simulink model "MCSI_simulation_2024_HDL_Coder_test"  (R2021a)
settings: Solver=VariableStepAuto  StartTime=0.0  StopTime=5/cfg.fl  FixedStep=2.0833e-8  RelTol=1e-3
undefined symbols (not defined in the file or in its folder): cfg
libraries: spsIdealSwitchLib x18, simulink x12, hdlsllib x8, spsSeriesRLCBranchLib x7, spsCurrentMeasurementLib x4, commutil2 x3, spsMeanLib x2, spsThreePhaseSeriesRLCBranchLib x2, spsThreePhaseVIMeasurementLib x2, spsControlledCurrentSourceLib x1, spsGroundLib x1, spsThreePhaseProgrammableGeneratorLib x1
settings Model: Creator=Damian  LastModifiedBy=Damian
settings SimscapeCC: SimscapeLogType=all  SimscapeLogLimitData=off

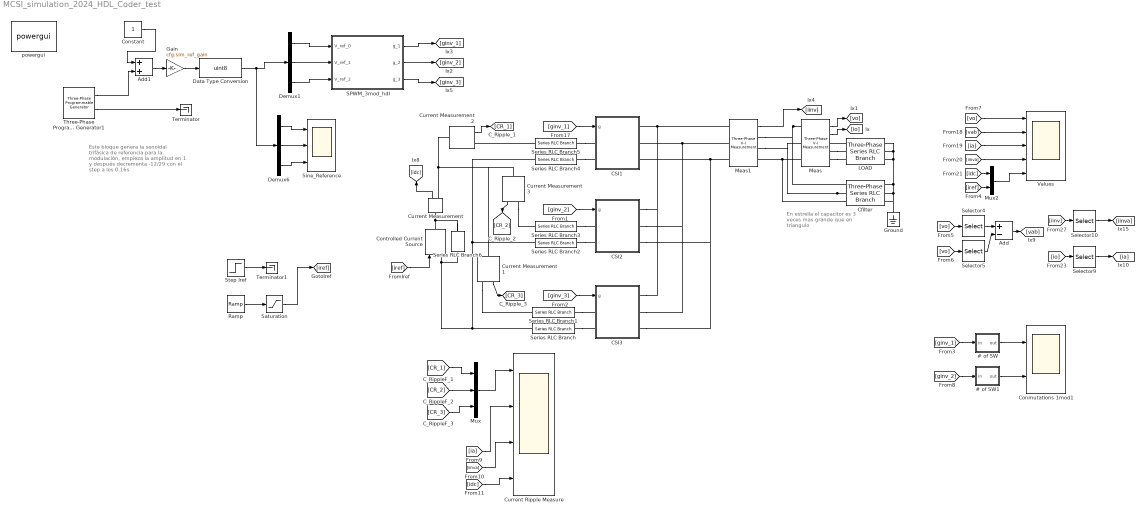
== system MCSI_simulation_2024_HDL_Coder_test ==
  note: Este bloque genera la senoidal
      | trifásica de referencia para la
      | modulación, empieza la amplitud
      | en 1 y después decrementa -12/29
      | con el step a los 0.16s
  note: En estrella el capacitor
      | es 3 veces mas grande
      | que en triangulo
  # of SW : Subsystem
  # of SW1 : Subsystem
  Add : Sum  Inputs=+-
  Add1 : Sum
  CSI1 : Subsystem
  CSI2 : Subsystem
  CSI3 : Subsystem
  Cfilter : spsThreePhaseSeriesRLCBranchLib/Three-Phase Series RLC Branch  LConnTagsString=A|B|C  RConnTagsString=A|B|C  BranchType=C  Resistance=1  Inductance=cfg.c  Capacitance=cfg.c  Measurements=None
  Conmutations 1mod1 : Scope  NumInputPorts=2
  Constant : Constant
  Controlled Current Source : spsControlledCurrentSourceLib/Controlled Current Source  Initialize=on  Source_Type=AC  Amplitude=0  Phase=0  Frequency=0  Measurements=None
  Current Measurement{,1..3} (4 alike) : spsCurrentMeasurementLib/Current Measurement  PhasorSimulation=off  OutputType=Complex  PSBequivalent=0
  Current Ripple Measure : Scope  NumInputPorts=4
  Data Type Conversion : DataTypeConversion  OutDataTypeStr=uint8
  Demux1 : Demux  Outputs=3
  Demux6 : Demux  Outputs=3
  Gain : Gain  Gain=cfg.sim_ref_gain
  Ground : spsGroundLib/Ground  LConnTagsString=a
  LOAD : spsThreePhaseSeriesRLCBranchLib/Three-Phase Series RLC Branch  LConnTagsString=A|B|C  RConnTagsString=A|B|C  BranchType=RL  Resistance=cfg.r  Inductance=cfg.l  Capacitance=1e-6  Measurements=None
  Meas : spsThreePhaseVIMeasurementLib/Three-Phase V-I Measurement  VoltageMeasurement=phase-to-ground  SetLabelV=off  LabelV=Vabc  Vpu=off  VpuLL=off  CurrentMeasurement=yes  SetLabelI=off  LabelI=Iabc  Ipu=off  Pbase=100e6  Vbase=500e3  OutputType=Complex  PhasorSimulation=off  PSBequivalent=0
  Meas1 : spsThreePhaseVIMeasurementLib/Three-Phase V-I Measurement  VoltageMeasurement=no  SetLabelV=off  LabelV=Vabc  Vpu=off  VpuLL=off  CurrentMeasurement=yes  SetLabelI=off  LabelI=Iabc  Ipu=off  Pbase=100e6  Vbase=500e3  OutputType=Complex  PhasorSimulation=off  PSBequivalent=0
  Mux : Mux  Inputs=3
  Mux2 : Mux  Inputs=2
  Ramp : simulink/Sources/Ramp  slope=cfg.iref/cfg.cs_soft_start_time  start=0  InitialOutput=0
  SPWM_3mod_hdl : Subsystem
  Saturation : Saturate  UpperLimit=10  LowerLimit=0
  Selector10 : Selector  InputPortWidth=3  IndexOptions=Index vector (dialog)  Indices=1  OutputSizes=1
  Selector4 : Selector  InputPortWidth=3  IndexOptions=Index vector (dialog)  Indices=1  OutputSizes=1
  Selector5 : Selector  InputPortWidth=3  IndexOptions=Index vector (dialog)  Indices=2  OutputSizes=1
  Selector9 : Selector  InputPortWidth=3  IndexOptions=Index vector (dialog)  Indices=1  OutputSizes=1
  Series RLC Branch{,1..5} (6 alike) : spsSeriesRLCBranchLib/Series RLC Branch  LConnTagsString=__new0  RConnTagsString=__new0  BranchType=L  Resistance=1  Inductance=cfg.sharing_L  SetiL0=off  InitialCurrent=0  Capacitance=1e-6  Setx0=off  InitialVoltage=0  Measurements=None
  Series RLC Branch6 : spsSeriesRLCBranchLib/Series RLC Branch  LConnTagsString=__new0  RConnTagsString=__new0  BranchType=R  Resistance=1E5  Inductance=cfg.sharing_L  SetiL0=off  InitialCurrent=0  Capacitance=1e-6  Setx0=off  InitialVoltage=0  Measurements=None
  Sine_Reference : Scope  NumInputPorts=3
  Step Iref : Step  Time=12/cfg.fl  Before=cfg.iref  After=0.6*cfg.iref  SampleTime=cfg.ts
  Terminator : Terminator
  Terminator1 : Terminator
  Three-Phase Programmable Generator1 : spsThreePhaseProgrammableGeneratorLib/Three-Phase Programmable Generator  Par_Vps=[1,-30, cfg.fl]  VariationEntity=None  VariationType=Step  VariationStep=-12/29  VariationRate=10  VariationMag=0.3  VariationFreq=2  Par_Timing_Variation="[8/cfg.fl  10]"  SinglePhase=on  Yampli=[1 0.2 1.2 1.0]  Xtime=[0 0.1 0.15 0.2]  HarmonicGeneration=off  Par_HarmoA="[3  5  -25 0]"  Par_HarmoB="[5  10  35  2]"  Par_Timing_Harmo="[ 0.05  99]"  Ts=cfg.ts
      settings: SourceProductBaseCode=PS
  Values : Scope  NumInputPorts=5
  powergui : spspowerguiLib/powergui  Priority=1  SimulationMode=Discrete  SampleTime=cfg.ts  frequency=60  Iterations=50  frequencyindice=0  Pbase=100e6  ErrMax=1e-4  UnitsV=kV  UnitsW=MW  buscounter=0  FunctionMessages=off  echomessages=off  EnableUseOfTLC=off  CurrentSourceSwitches=off  DisableSnubberDevices=off  DisableRonSwitches=off  DisableVfSwitches=off  DisplayEquations=off  AutomaticDiscreteSolvers=off  SolverType=Backward Euler  Interpol=off  ExternalGateDelay=off  methode=off  Ts=0  x0status=blocks  SPID=off  SwTol=0  HookPort=off  NonlinearTolerance=1e-4  nMaxIteration=100  ContinueOnMaxIteration=off  RestoreLinks=warning  ResistiveCurrentMeasurement=off  Frange=[0:2:500]  Ylog=off  Xlog=on  ShowGrid=off  save=off  variable=ZData  structure=one_mod_model  ZoomFFT=off  StartTime=0.12  cycles=1  DisplayStyle=1  fundamental=50  FreqAxis=off  MaxFrequency=1000  frequencyindicesteady=1  RmsSteady=1  display=off
  wires:
  [iref] -> Controlled Current Source/1
  Current Measurement/1 -> [idc]
  Three-Phase Programmable Generator1/2 -> Terminator/1
  Three-Phase Programmable Generator1/1 -> Add1/2
  Demux6/3 -> Sine_Reference/3
  Demux6/2 -> Sine_Reference/2
  Demux6/1 -> Sine_Reference/1
  [ginv_1] -> CSI1/1(g)
  Meas/1 -> [vo]
  Meas/2 -> [io]
  Meas1/1 -> [iinv]
  [iref] -> Mux2/2
  [idc] -> Mux2/1
  Mux2/1 -> Values/5
  [vo] -> Values/1
  [iinva] -> Values/4
  [ia] -> Values/3
  [vab] -> Values/2
  [vo] -> Selector4/1
  [vo] -> Selector5/1
  Selector4/1 -> Add/1
  Selector5/1 -> Add/2
  Add/1 -> [vab]
  [iinv] -> Selector10/1
  [io] -> Selector9/1
  Selector10/1 -> [iinva]
  Selector9/1 -> [ia]
  [ginv_2] -> CSI2/1(g)
  [ginv_3] -> CSI3/1(g)
  [ginv_1] -> # of SW/1(in)
  # of SW/1(out) -> Conmutations 1mod1/1
  # of SW1/1(out) -> Conmutations 1mod1/2
  [ginv_2] -> # of SW1/1(in)
  Saturation/1 -> [iref]
  Ramp/1 -> Saturation/1
  Step Iref/1 -> Terminator1/1
  Current Measurement2/1 -> [CR_1]
  Current Measurement3/1 -> [CR_2]
  Current Measurement1/1 -> [CR_3]
  [ia] -> Current Ripple Measure/2
  [iinva] -> Current Ripple Measure/3
  [idc] -> Current Ripple Measure/4
  [CR_1] -> Mux/1
  [CR_2] -> Mux/2
  [CR_3] -> Mux/3
  Mux/1 -> Current Ripple Measure/1
  Constant/1 -> Add1/1
  Add1/1 -> Gain/1
  Gain/1 -> Data Type Conversion/1
  Data Type Conversion/1 -> Demux6/1, Demux1/1
  Demux1/3 -> SPWM_3mod_hdl/3(V_ref_2)
  Demux1/2 -> SPWM_3mod_hdl/2(V_ref_1)
  Demux1/1 -> SPWM_3mod_hdl/1(V_ref_0)
  SPWM_3mod_hdl/1(g_1) -> [ginv_1]
  SPWM_3mod_hdl/2(g_2) -> [ginv_2]
  SPWM_3mod_hdl/3(g_3) -> [ginv_3]
  connections:
  Current Measurement/LConn1 -- Series RLC Branch6/LConn1 -- Controlled Current Source/RConn1
  Meas/LConn3 -- Cfilter/LConn3 -- Meas1/RConn3
  Meas/LConn1 -- Meas1/RConn1 -- Cfilter/LConn1
  LOAD/RConn2 -- LOAD/RConn1 -- LOAD/RConn3 -- Cfilter/RConn1 -- Cfilter/RConn2 -- Cfilter/RConn3 -- Ground/LConn1
  Cfilter/LConn2 -- Meas1/RConn2 -- Meas/LConn2
  LOAD/LConn1 -- Meas/RConn1
  Meas/RConn2 -- LOAD/LConn2
  Meas/RConn3 -- LOAD/LConn3
  Meas1/LConn1 -- CSI3/RConn1 -- CSI2/RConn1 -- CSI1/RConn1
  Meas1/LConn2 -- CSI3/RConn2 -- CSI2/RConn2 -- CSI1/RConn2
  Meas1/LConn3 -- CSI3/RConn3 -- CSI2/RConn3 -- CSI1/RConn3
  Series RLC Branch4/RConn1 -- CSI1/LConn2
  Series RLC Branch5/RConn1 -- CSI1/LConn1
  Series RLC Branch3/RConn1 -- CSI2/LConn1
  Series RLC Branch2/RConn1 -- CSI2/LConn2
  Series RLC Branch1/RConn1 -- CSI3/LConn1
  Series RLC Branch/RConn1 -- CSI3/LConn2
  Controlled Current Source/LConn1 -- Series RLC Branch/LConn1 -- Series RLC Branch2/LConn1 -- Series RLC Branch4/LConn1 -- Series RLC Branch6/RConn1
  Current Measurement3/RConn1 -- Series RLC Branch3/LConn1
  Current Measurement2/LConn1 -- Current Measurement3/LConn1 -- Current Measurement1/LConn1 -- Current Measurement/RConn1
  Current Measurement1/RConn1 -- Series RLC Branch1/LConn1
  Series RLC Branch5/LConn1 -- Current Measurement2/RConn1

== system MCSI_simulation_2024_HDL_Coder_test/# of SW ==
  in : Inport
  Data Type Conversion : DataTypeConversion
  Detect Change : simulink/Logic and Bit Operations/Detect Change  vinit=0  OutDataTypeStr=boolean
  Divide : Product  Inputs=*/
  Gain : Gain  Gain=1/cfg.ts
  Mean1 : spsMeanLib/Mean  Freq=cfg.fl  Vinit=0  Ts=cfg.ts
  Sum of Elements : Sum  Inputs=+
  Width : Width
  out : Outport
  wires:
  Detect Change/1 -> Data Type Conversion/1
  Mean1/1 -> Gain/1
  Data Type Conversion/1 -> Mean1/1
  in/1 -> Detect Change/1
  Gain/1 -> Width/1, Sum of Elements/1
  Sum of Elements/1 -> Divide/1
  Width/1 -> Divide/2
  Divide/1 -> out/1

== system MCSI_simulation_2024_HDL_Coder_test/# of SW1 ==
  in : Inport
  Data Type Conversion : DataTypeConversion
  Detect Change : simulink/Logic and Bit Operations/Detect Change  vinit=0  OutDataTypeStr=boolean
  Gain : Gain  Gain=1/cfg.ts
  Mean1 : spsMeanLib/Mean  Freq=cfg.fl  Vinit=0  Ts=cfg.ts
  out : Outport
  wires:
  Detect Change/1 -> Data Type Conversion/1
  Mean1/1 -> Gain/1
  Data Type Conversion/1 -> Mean1/1
  in/1 -> Detect Change/1
  Gain/1 -> out/1

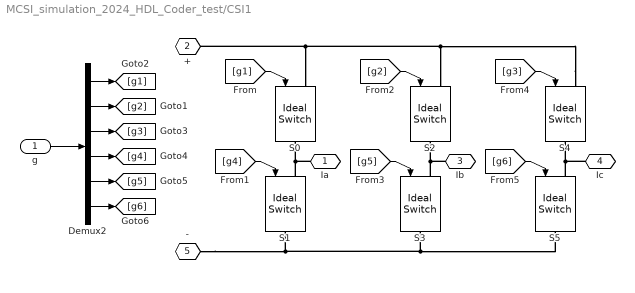
== system MCSI_simulation_2024_HDL_Coder_test/CSI1 ==
  g : Inport
  Demux2 : Demux  Outputs=6
  S{0..5} (6 alike) : spsIdealSwitchLib/Ideal Switch  Ron=cfg.switch.Ron  Lon=0  IC=0  Rs=cfg.switch.snubber_Rs  Cs=cfg.switch.snubber_Cs  Measurements=off
  Ia : PMIOPort  Side=Right
  + : PMIOPort  Port=2  Side=Left
  Ib : PMIOPort  Port=3  Side=Right
  Ic : PMIOPort  Port=4  Side=Right
  - : PMIOPort  Port=5  Side=Left
  wires:
  Demux2/1 -> [g1]
  Demux2/4 -> [g4]
  g/1 -> Demux2/1
  [g4] -> S1/1
  [g2] -> S2/1
  [g5] -> S3/1
  Demux2/5 -> [g5]
  [g3] -> S4/1
  [g6] -> S5/1
  Demux2/6 -> [g6]
  Demux2/3 -> [g3]
  Demux2/2 -> [g2]
  [g1] -> S0/1
  connections:
  S1/LConn1 -- Ia/RConn1 -- S0/RConn1
  S3/LConn1 -- Ib/RConn1 -- S2/RConn1
  S5/LConn1 -- Ic/RConn1 -- S4/RConn1
  S4/LConn1 -- S2/LConn1 -- S0/LConn1 -- +/RConn1
  -/RConn1 -- S5/RConn1 -- S3/RConn1 -- S1/RConn1

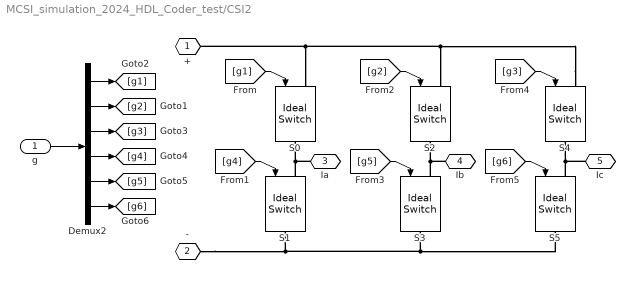
== system MCSI_simulation_2024_HDL_Coder_test/CSI2 ==
  g : Inport
  Demux2 : Demux  Outputs=6
  S{0..5} (6 alike) : spsIdealSwitchLib/Ideal Switch  Ron=cfg.switch.Ron  Lon=0  IC=0  Rs=cfg.switch.snubber_Rs  Cs=cfg.switch.snubber_Cs  Measurements=off
  + : PMIOPort  Side=Left
  - : PMIOPort  Port=2  Side=Left
  Ia : PMIOPort  Port=3  Side=Right
  Ib : PMIOPort  Port=4  Side=Right
  Ic : PMIOPort  Port=5  Side=Right
  wires:
  Demux2/1 -> [g1]
  Demux2/4 -> [g4]
  g/1 -> Demux2/1
  [g4] -> S1/1
  [g2] -> S2/1
  [g5] -> S3/1
  Demux2/5 -> [g5]
  [g3] -> S4/1
  [g6] -> S5/1
  Demux2/6 -> [g6]
  Demux2/3 -> [g3]
  Demux2/2 -> [g2]
  [g1] -> S0/1
  connections:
  S1/LConn1 -- Ia/RConn1 -- S0/RConn1
  S3/LConn1 -- Ib/RConn1 -- S2/RConn1
  S5/LConn1 -- Ic/RConn1 -- S4/RConn1
  S4/LConn1 -- S2/LConn1 -- S0/LConn1 -- +/RConn1
  -/RConn1 -- S5/RConn1 -- S3/RConn1 -- S1/RConn1

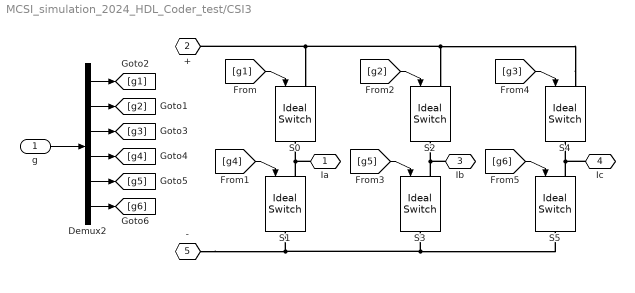
== system MCSI_simulation_2024_HDL_Coder_test/CSI3 ==
  g : Inport
  Demux2 : Demux  Outputs=6
  S{0..5} (6 alike) : spsIdealSwitchLib/Ideal Switch  Ron=cfg.switch.Ron  Lon=0  IC=0  Rs=cfg.switch.snubber_Rs  Cs=cfg.switch.snubber_Cs  Measurements=off
  Ia : PMIOPort  Side=Right
  + : PMIOPort  Port=2  Side=Left
  Ib : PMIOPort  Port=3  Side=Right
  Ic : PMIOPort  Port=4  Side=Right
  - : PMIOPort  Port=5  Side=Left
  wires:
  Demux2/1 -> [g1]
  Demux2/4 -> [g4]
  g/1 -> Demux2/1
  [g4] -> S1/1
  [g2] -> S2/1
  [g5] -> S3/1
  Demux2/5 -> [g5]
  [g3] -> S4/1
  [g6] -> S5/1
  Demux2/6 -> [g6]
  Demux2/3 -> [g3]
  Demux2/2 -> [g2]
  [g1] -> S0/1
  connections:
  S1/LConn1 -- Ia/RConn1 -- S0/RConn1
  S3/LConn1 -- Ib/RConn1 -- S2/RConn1
  S5/LConn1 -- Ic/RConn1 -- S4/RConn1
  S4/LConn1 -- S2/LConn1 -- S0/LConn1 -- +/RConn1
  -/RConn1 -- S5/RConn1 -- S3/RConn1 -- S1/RConn1

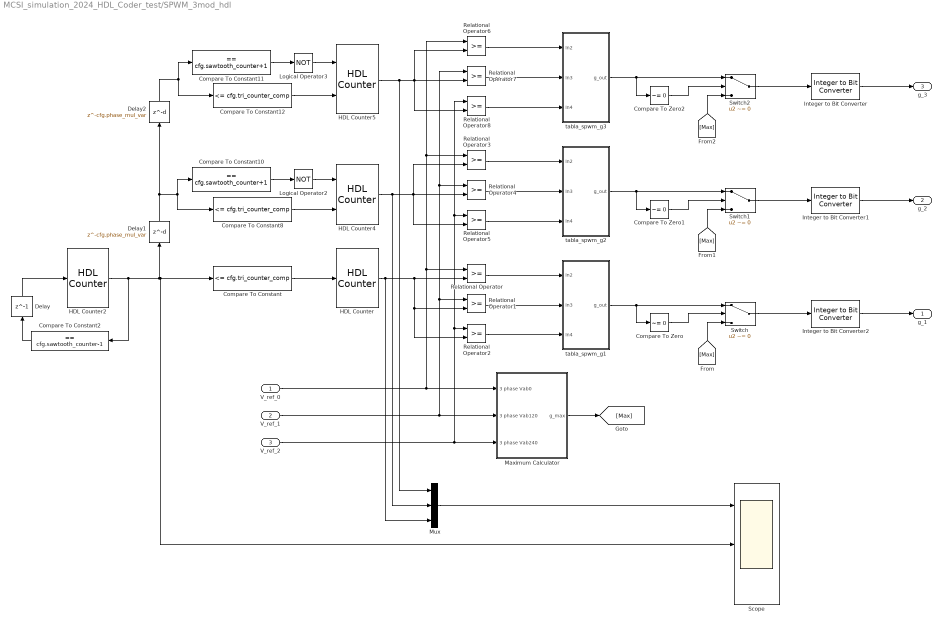
== system MCSI_simulation_2024_HDL_Coder_test/SPWM_3mod_hdl ==
  V_ref_0 : Inport  OutDataTypeStr=fixdt(0,8,0)
  V_ref_1 : Inport  Port=2  OutDataTypeStr=fixdt(0,8,0)
  V_ref_2 : Inport  Port=3  OutDataTypeStr=fixdt(0,8,0)
  Compare To Constant : simulink/Logic and Bit Operations/Compare To Constant  relop=<=  const=cfg.tri_counter_comp  OutDataTypeStr=boolean
  Compare To Constant10 : simulink/Logic and Bit Operations/Compare To Constant  relop===  const=cfg.sawtooth_counter+1  OutDataTypeStr=boolean
  Compare To Constant11 : simulink/Logic and Bit Operations/Compare To Constant  relop===  const=cfg.sawtooth_counter+1  OutDataTypeStr=boolean
  Compare To Constant12 : simulink/Logic and Bit Operations/Compare To Constant  relop=<=  const=cfg.tri_counter_comp  OutDataTypeStr=boolean
  Compare To Constant2 : simulink/Logic and Bit Operations/Compare To Constant  relop===  const=cfg.sawtooth_counter-1  OutDataTypeStr=boolean
  Compare To Constant8 : simulink/Logic and Bit Operations/Compare To Constant  relop=<=  const=cfg.tri_counter_comp  OutDataTypeStr=boolean
  Compare To Zero : simulink/Logic and Bit Operations/Compare To Zero  relop=~=  OutDataTypeStr=boolean
  Compare To Zero1 : simulink/Logic and Bit Operations/Compare To Zero  relop=~=  OutDataTypeStr=boolean
  Compare To Zero2 : simulink/Logic and Bit Operations/Compare To Zero  relop=~=  OutDataTypeStr=boolean
  Delay : Delay  DelayLength=1  InitialCondition=0
  Delay1 : Delay  DelayLength=cfg.phase_mul_var  InitialCondition=cfg.sawtooth_counter+1
  Delay2 : Delay  DelayLength=cfg.phase_mul_var  InitialCondition=cfg.sawtooth_counter+1
  HDL Counter : hdlsllib/Sources/HDL Counter  CountType=Free running  CountInit=0  CountStep=1  CountMax=255  CountFromType=Initial value  CountFrom=0  CountResetPort=off  CountLoadPort=off  CountEnbPort=off  CountDirPort=on  CountHitOutputPort=off  CountDataType=Unsigned  CountWordLen=cfg.counter_tri_word_length  CountFracLen=0  CountSampTime=1
  HDL Counter2 : hdlsllib/Sources/HDL Counter  CountType=Free running  CountInit=0  CountStep=1  CountMax=cfg.sawtooth_counter-1  CountFromType=Initial value  CountFrom=0  CountResetPort=on  CountLoadPort=off  CountEnbPort=off  CountDirPort=off  CountHitOutputPort=off  CountDataType=Unsigned  CountWordLen=cfg.counter_word_length  CountFracLen=0  CountSampTime=1
  HDL Counter4 : hdlsllib/Sources/HDL Counter  CountType=Free running  CountInit=0  CountStep=1  CountMax=255  CountFromType=Initial value  CountFrom=0  CountResetPort=off  CountLoadPort=off  CountEnbPort=on  CountDirPort=on  CountHitOutputPort=off  CountDataType=Unsigned  CountWordLen=cfg.counter_tri_word_length  CountFracLen=0  CountSampTime=1
  HDL Counter5 : hdlsllib/Sources/HDL Counter  CountType=Free running  CountInit=0  CountStep=1  CountMax=255  CountFromType=Initial value  CountFrom=0  CountResetPort=off  CountLoadPort=off  CountEnbPort=on  CountDirPort=on  CountHitOutputPort=off  CountDataType=Unsigned  CountWordLen=cfg.counter_tri_word_length  CountFracLen=0  CountSampTime=1
  Integer to Bit Converter : commutil2/Integer to Bit Converter  nbits=6  signedInputValues=Unsigned  bitOrder=MSB first  outDtype=Inherit via internal rule
  Integer to Bit Converter1 : commutil2/Integer to Bit Converter  nbits=6  signedInputValues=Unsigned  bitOrder=MSB first  outDtype=Inherit via internal rule
  Integer to Bit Converter2 : commutil2/Integer to Bit Converter  nbits=6  signedInputValues=Unsigned  bitOrder=MSB first  outDtype=Inherit via internal rule
  Logical Operator2 : Logic  Operator=NOT  AllPortsSameDT=off  OutDataTypeStr=boolean
  Logical Operator3 : Logic  Operator=NOT  AllPortsSameDT=off  OutDataTypeStr=boolean
  Maximum Calculator : Subsystem
  Mux : Mux  Inputs=3
  Relational Operator{,1..8} (9 alike) : RelationalOperator  OutDataTypeStr=boolean  RndMeth=Nearest
  Scope : Scope  NumInputPorts=3
  Switch : Switch  Criteria=u2 ~= 0
  Switch1 : Switch  Criteria=u2 ~= 0
  Switch2 : Switch  Criteria=u2 ~= 0
  tabla_spwm_g1 : Subsystem
  tabla_spwm_g2 : Subsystem
  tabla_spwm_g3 : Subsystem
  g_1 : Outport
  g_2 : Outport  Port=2
  g_3 : Outport  Port=3
  wires:
  HDL Counter4/1 -> Relational Operator4/2, Relational Operator3/2, Relational Operator5/2, Mux/2
  Compare To Constant12/1 -> HDL Counter5/2
  tabla_spwm_g3/1(g_out) -> Compare To Zero2/1, Switch2/1
  V_ref_2/1 -> Relational Operator5/1, Relational Operator8/1, Relational Operator2/1, Maximum Calculator/3(3 phase Vab240)
  Delay1/1 -> Delay2/1, Compare To Constant10/1, Compare To Constant8/1
  [Max] -> Switch/3
  Relational Operator1/1 -> tabla_spwm_g1/2(In3)
  Delay2/1 -> Compare To Constant11/1, Compare To Constant12/1
  tabla_spwm_g1/1(g_out) -> Compare To Zero/1, Switch/1
  Relational Operator/1 -> tabla_spwm_g1/1(In2)
  Relational Operator7/1 -> tabla_spwm_g3/2(In3)
  Logical Operator2/1 -> HDL Counter4/1
  Relational Operator8/1 -> tabla_spwm_g3/3(In4)
  Delay/1 -> HDL Counter2/1
  V_ref_1/1 -> Maximum Calculator/2(3 phase Vab120), Relational Operator1/1, Relational Operator4/1, Relational Operator7/1
  Compare To Zero2/1 -> Switch2/2
  V_ref_0/1 -> Maximum Calculator/1(3 phase Vab0), Relational Operator/1, Relational Operator3/1, Relational Operator6/1
  Compare To Constant2/1 -> Delay/1
  [Max] -> Switch2/3
  Maximum Calculator/1(g_max) -> [Max]
  Relational Operator6/1 -> tabla_spwm_g3/1(In2)
  HDL Counter2/1 -> Compare To Constant2/1, Delay1/1, Scope/2, Compare To Constant/1
  HDL Counter5/1 -> Relational Operator7/2, Relational Operator6/2, Relational Operator8/2, Mux/1
  HDL Counter/1 -> Mux/3, Relational Operator2/2, Relational Operator1/2, Relational Operator/2
  Compare To Constant10/1 -> Logical Operator2/1
  Compare To Zero/1 -> Switch/2
  Relational Operator5/1 -> tabla_spwm_g2/3(In4)
  Relational Operator2/1 -> tabla_spwm_g1/3(In4)
  Compare To Constant/1 -> HDL Counter/1
  tabla_spwm_g2/1(g_out) -> Compare To Zero1/1, Switch1/1
  [Max] -> Switch1/3
  Compare To Constant8/1 -> HDL Counter4/2
  Compare To Constant11/1 -> Logical Operator3/1
  Compare To Zero1/1 -> Switch1/2
  Logical Operator3/1 -> HDL Counter5/1
  Relational Operator3/1 -> tabla_spwm_g2/1(In2)
  Relational Operator4/1 -> tabla_spwm_g2/2(In3)
  Switch/1 -> Integer to Bit Converter2/1
  Integer to Bit Converter2/1 -> g_1/1
  Switch1/1 -> Integer to Bit Converter1/1
  Integer to Bit Converter1/1 -> g_2/1
  Switch2/1 -> Integer to Bit Converter/1
  Integer to Bit Converter/1 -> g_3/1
  Mux/1 -> Scope/1

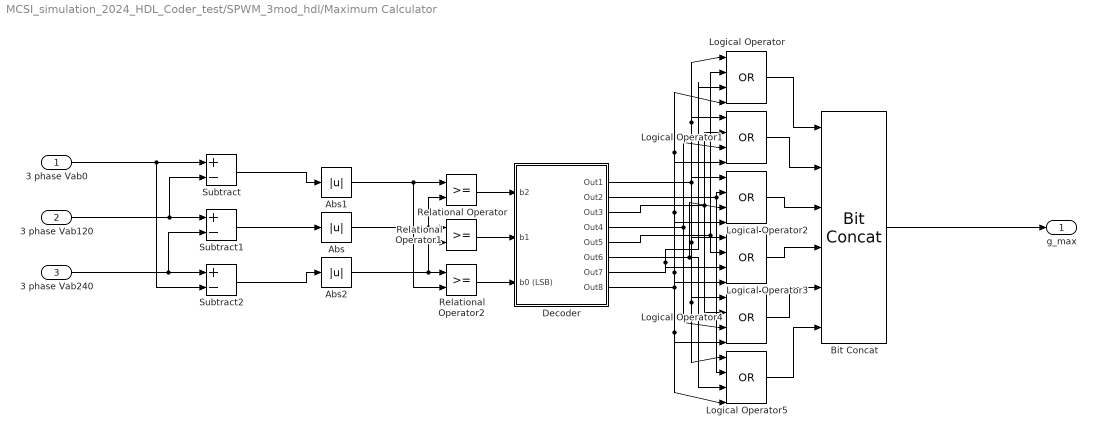
== system MCSI_simulation_2024_HDL_Coder_test/SPWM_3mod_hdl/Maximum Calculator ==
  3 phase Vab0 : Inport
  3 phase Vab120 : Inport  Port=2
  3 phase Vab240 : Inport  Port=3
  Abs : Abs
  Abs1 : Abs
  Abs2 : Abs
  Bit Concat : hdlsllib/Logic and Bit Operations/Bit Concat  numInputs=6
  Decoder : Subsystem
  Logical Operator{,1..5} (6 alike) : Logic  Operator=OR  Inputs=4  IconShape=distinctive  AllPortsSameDT=off  OutDataTypeStr=boolean
  Relational Operator : RelationalOperator  OutDataTypeStr=boolean  RndMeth=Nearest
  Relational Operator1 : RelationalOperator  OutDataTypeStr=boolean  RndMeth=Nearest
  Relational Operator2 : RelationalOperator  OutDataTypeStr=boolean  RndMeth=Nearest
  Subtract : Sum  Inputs=+-  OutDataTypeStr=int32
  Subtract1 : Sum  Inputs=+-  OutDataTypeStr=int32
  Subtract2 : Sum  Inputs=+-  OutDataTypeStr=int32
  g_max : Outport  VectorParamsAs1DForOutWhenUnconnected=off
  wires:
  Relational Operator/1 -> Decoder/1(b2)
  Abs1/1 -> Relational Operator/1, Relational Operator2/2
  Logical Operator2/1 -> Bit Concat/3
  Abs/1 -> Relational Operator/2, Relational Operator1/1
  3 phase Vab0/1 -> Subtract2/2, Subtract/1
  Decoder/6(Out6) -> Logical Operator5/3, Logical Operator2/3
  Decoder/3(Out3) -> Logical Operator4/2, Logical Operator1/2
  Decoder/2(Out2) -> Logical Operator2/2, Logical Operator5/2
  3 phase Vab240/1 -> Subtract2/1, Subtract1/2
  Logical Operator5/1 -> Bit Concat/6
  Decoder/1(Out1) -> Logical Operator1/1, Logical Operator/1, Logical Operator5/1, Logical Operator4/1, Logical Operator3/1, Logical Operator2/1
  Abs2/1 -> Relational Operator1/2, Relational Operator2/1
  Subtract1/1 -> Abs/1
  Decoder/4(Out4) -> Logical Operator4/3, Logical Operator1/3
  3 phase Vab120/1 -> Subtract1/1, Subtract/2
  Logical Operator3/1 -> Bit Concat/4
  Decoder/5(Out5) -> Logical Operator3/2, Logical Operator/2
  Subtract/1 -> Abs1/1
  Subtract2/1 -> Abs2/1
  Relational Operator1/1 -> Decoder/2(b1)
  Relational Operator2/1 -> Decoder/3(b0 (LSB))
  Logical Operator1/1 -> Bit Concat/2
  Decoder/8(Out8) -> Logical Operator/4, Logical Operator1/4, Logical Operator2/4, Logical Operator3/4, Logical Operator4/4, Logical Operator5/4
  Decoder/7(Out7) -> Logical Operator3/3, Logical Operator/3
  Logical Operator4/1 -> Bit Concat/5
  Logical Operator/1 -> Bit Concat/1
  Bit Concat/1 -> g_max/1

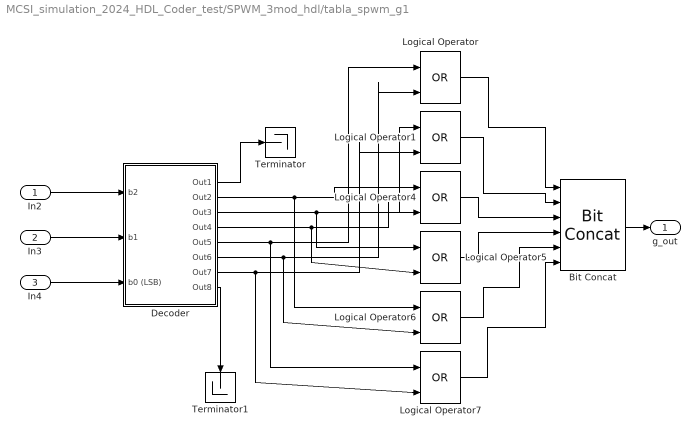
== system MCSI_simulation_2024_HDL_Coder_test/SPWM_3mod_hdl/tabla_spwm_g1 ==
  In2 : Inport
  In3 : Inport  Port=2
  In4 : Inport  Port=3
  Bit Concat : hdlsllib/Logic and Bit Operations/Bit Concat  numInputs=6
  Decoder : Subsystem
  Logical Operator{,1,4..7} (6 alike) : Logic  Operator=OR  IconShape=distinctive  AllPortsSameDT=off  OutDataTypeStr=boolean
  Terminator : Terminator
  Terminator1 : Terminator
  g_out : Outport  VectorParamsAs1DForOutWhenUnconnected=off
  wires:
  Decoder/7(Out7) -> Logical Operator1/2, Logical Operator7/2
  Logical Operator4/1 -> Bit Concat/3
  Logical Operator/1 -> Bit Concat/1
  Logical Operator1/1 -> Bit Concat/2
  Decoder/2(Out2) -> Logical Operator4/1, Logical Operator6/1
  Logical Operator7/1 -> Bit Concat/6
  Logical Operator5/1 -> Bit Concat/4
  Decoder/5(Out5) -> Logical Operator/1, Logical Operator7/1
  Logical Operator6/1 -> Bit Concat/5
  In4/1 -> Decoder/3(b0 (LSB))
  In3/1 -> Decoder/2(b1)
  In2/1 -> Decoder/1(b2)
  Decoder/4(Out4) -> Logical Operator5/2, Logical Operator4/2
  Decoder/3(Out3) -> Logical Operator5/1, Logical Operator1/1
  Decoder/6(Out6) -> Logical Operator/2, Logical Operator6/2
  Decoder/1(Out1) -> Terminator/1
  Decoder/8(Out8) -> Terminator1/1
  Bit Concat/1 -> g_out/1

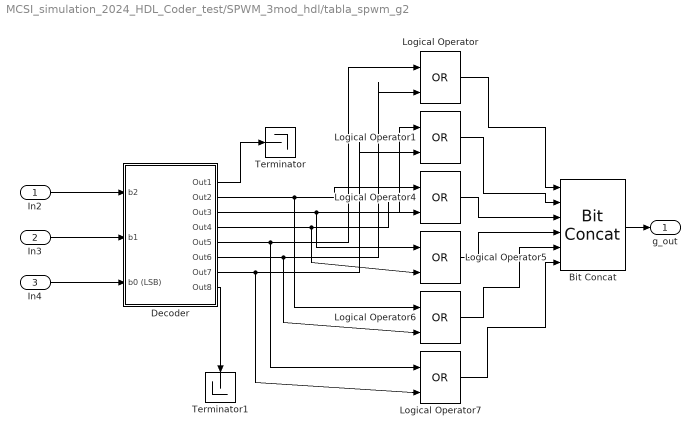
== system MCSI_simulation_2024_HDL_Coder_test/SPWM_3mod_hdl/tabla_spwm_g2 ==
  In2 : Inport
  In3 : Inport  Port=2
  In4 : Inport  Port=3
  Bit Concat : hdlsllib/Logic and Bit Operations/Bit Concat  numInputs=6
  Decoder : Subsystem
  Logical Operator{,1,4..7} (6 alike) : Logic  Operator=OR  IconShape=distinctive  AllPortsSameDT=off  OutDataTypeStr=boolean
  Terminator : Terminator
  Terminator1 : Terminator
  g_out : Outport  VectorParamsAs1DForOutWhenUnconnected=off
  wires:
  Decoder/7(Out7) -> Logical Operator1/2, Logical Operator7/2
  Logical Operator4/1 -> Bit Concat/3
  Logical Operator/1 -> Bit Concat/1
  Logical Operator1/1 -> Bit Concat/2
  Decoder/2(Out2) -> Logical Operator4/1, Logical Operator6/1
  Logical Operator7/1 -> Bit Concat/6
  Logical Operator5/1 -> Bit Concat/4
  Decoder/5(Out5) -> Logical Operator/1, Logical Operator7/1
  Logical Operator6/1 -> Bit Concat/5
  In4/1 -> Decoder/3(b0 (LSB))
  In3/1 -> Decoder/2(b1)
  In2/1 -> Decoder/1(b2)
  Decoder/4(Out4) -> Logical Operator5/2, Logical Operator4/2
  Decoder/3(Out3) -> Logical Operator5/1, Logical Operator1/1
  Decoder/6(Out6) -> Logical Operator/2, Logical Operator6/2
  Decoder/1(Out1) -> Terminator/1
  Decoder/8(Out8) -> Terminator1/1
  Bit Concat/1 -> g_out/1

== system MCSI_simulation_2024_HDL_Coder_test/SPWM_3mod_hdl/tabla_spwm_g3 ==
  In2 : Inport
  In3 : Inport  Port=2
  In4 : Inport  Port=3
  Bit Concat : hdlsllib/Logic and Bit Operations/Bit Concat  numInputs=6
  Decoder : Subsystem
  Logical Operator{,1,4..7} (6 alike) : Logic  Operator=OR  IconShape=distinctive  AllPortsSameDT=off  OutDataTypeStr=boolean
  Terminator : Terminator
  Terminator1 : Terminator
  g_out : Outport  VectorParamsAs1DForOutWhenUnconnected=off
  wires:
  Decoder/7(Out7) -> Logical Operator1/2, Logical Operator7/2
  Logical Operator4/1 -> Bit Concat/3
  Logical Operator/1 -> Bit Concat/1
  Logical Operator1/1 -> Bit Concat/2
  Decoder/2(Out2) -> Logical Operator4/1, Logical Operator6/1
  Logical Operator7/1 -> Bit Concat/6
  Logical Operator5/1 -> Bit Concat/4
  Decoder/5(Out5) -> Logical Operator/1, Logical Operator7/1
  Logical Operator6/1 -> Bit Concat/5
  In4/1 -> Decoder/3(b0 (LSB))
  In3/1 -> Decoder/2(b1)
  In2/1 -> Decoder/1(b2)
  Decoder/4(Out4) -> Logical Operator5/2, Logical Operator4/2
  Decoder/3(Out3) -> Logical Operator5/1, Logical Operator1/1
  Decoder/6(Out6) -> Logical Operator/2, Logical Operator6/2
  Decoder/1(Out1) -> Terminator/1
  Decoder/8(Out8) -> Terminator1/1
  Bit Concat/1 -> g_out/1

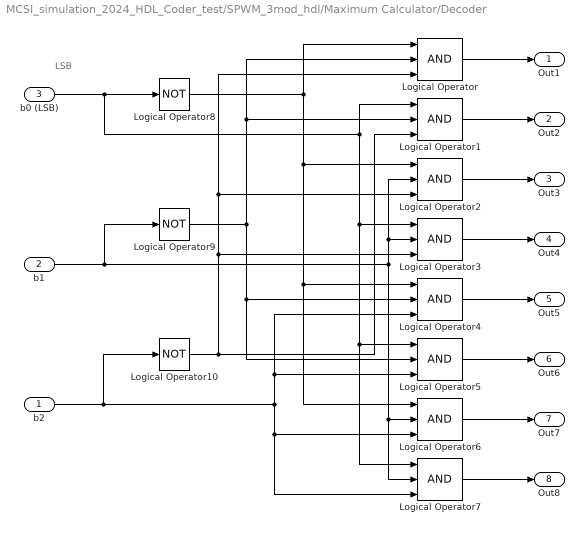
== system MCSI_simulation_2024_HDL_Coder_test/SPWM_3mod_hdl/Maximum Calculator/Decoder ==
  note: LSB
  b2 : Inport
  b1 : Inport  Port=2
  b0 (LSB) : Inport  Port=3
  Logical Operator{,1..7} (8 alike) : Logic  Inputs=3  IconShape=distinctive  AllPortsSameDT=off  OutDataTypeStr=boolean
  Logical Operator10 : Logic  Operator=NOT  IconShape=distinctive  AllPortsSameDT=off  OutDataTypeStr=boolean
  Logical Operator8 : Logic  Operator=NOT  IconShape=distinctive  AllPortsSameDT=off  OutDataTypeStr=boolean
  Logical Operator9 : Logic  Operator=NOT  IconShape=distinctive  AllPortsSameDT=off  OutDataTypeStr=boolean
  Out1 : Outport
  Out2 : Outport  Port=2
  Out3 : Outport  Port=3
  Out4 : Outport  Port=4
  Out5 : Outport  Port=5
  Out6 : Outport  Port=6
  Out7 : Outport  Port=7
  Out8 : Outport  Port=8
  wires:
  Logical Operator9/1 -> Logical Operator5/2, Logical Operator4/2, Logical Operator1/2, Logical Operator/2
  Logical Operator5/1 -> Out6/1
  Logical Operator1/1 -> Out2/1
  Logical Operator10/1 -> Logical Operator3/3, Logical Operator2/3, Logical Operator/3, Logical Operator1/3
  Logical Operator/1 -> Out1/1
  Logical Operator8/1 -> Logical Operator6/1, Logical Operator4/1, Logical Operator2/1, Logical Operator/1
  b2/1 -> Logical Operator4/3, Logical Operator5/3, Logical Operator7/3, Logical Operator6/3, Logical Operator10/1
  b0 (LSB)/1 -> Logical Operator7/1, Logical Operator5/1, Logical Operator3/1, Logical Operator1/1, Logical Operator8/1
  Logical Operator7/1 -> Out8/1
  b1/1 -> Logical Operator3/2, Logical Operator2/2, Logical Operator7/2, Logical Operator6/2, Logical Operator9/1
  Logical Operator4/1 -> Out5/1
  Logical Operator6/1 -> Out7/1
  Logical Operator3/1 -> Out4/1
  Logical Operator2/1 -> Out3/1

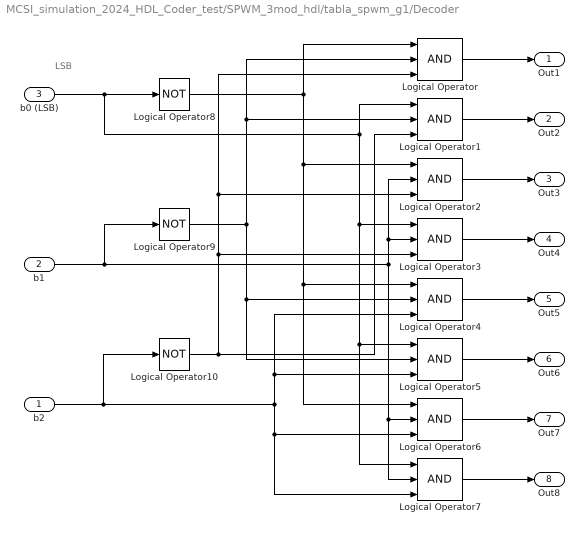
== system MCSI_simulation_2024_HDL_Coder_test/SPWM_3mod_hdl/tabla_spwm_g1/Decoder ==
  note: LSB
  b2 : Inport
  b1 : Inport  Port=2
  b0 (LSB) : Inport  Port=3
  Logical Operator{,1..7} (8 alike) : Logic  Inputs=3  IconShape=distinctive  AllPortsSameDT=off  OutDataTypeStr=boolean
  Logical Operator10 : Logic  Operator=NOT  IconShape=distinctive  AllPortsSameDT=off  OutDataTypeStr=boolean
  Logical Operator8 : Logic  Operator=NOT  IconShape=distinctive  AllPortsSameDT=off  OutDataTypeStr=boolean
  Logical Operator9 : Logic  Operator=NOT  IconShape=distinctive  AllPortsSameDT=off  OutDataTypeStr=boolean
  Out1 : Outport
  Out2 : Outport  Port=2
  Out3 : Outport  Port=3
  Out4 : Outport  Port=4
  Out5 : Outport  Port=5
  Out6 : Outport  Port=6
  Out7 : Outport  Port=7
  Out8 : Outport  Port=8
  wires:
  Logical Operator9/1 -> Logical Operator5/2, Logical Operator4/2, Logical Operator1/2, Logical Operator/2
  Logical Operator5/1 -> Out6/1
  Logical Operator1/1 -> Out2/1
  Logical Operator10/1 -> Logical Operator3/3, Logical Operator2/3, Logical Operator/3, Logical Operator1/3
  Logical Operator/1 -> Out1/1
  Logical Operator8/1 -> Logical Operator6/1, Logical Operator4/1, Logical Operator2/1, Logical Operator/1
  b2/1 -> Logical Operator4/3, Logical Operator5/3, Logical Operator7/3, Logical Operator6/3, Logical Operator10/1
  b0 (LSB)/1 -> Logical Operator7/1, Logical Operator5/1, Logical Operator3/1, Logical Operator1/1, Logical Operator8/1
  Logical Operator7/1 -> Out8/1
  b1/1 -> Logical Operator3/2, Logical Operator2/2, Logical Operator7/2, Logical Operator6/2, Logical Operator9/1
  Logical Operator4/1 -> Out5/1
  Logical Operator6/1 -> Out7/1
  Logical Operator3/1 -> Out4/1
  Logical Operator2/1 -> Out3/1

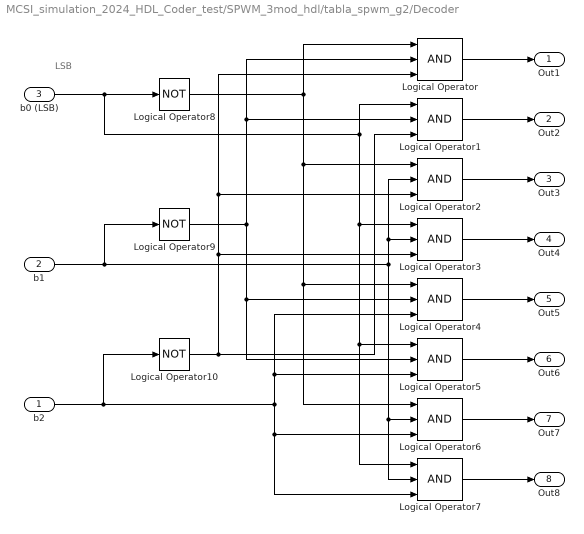
== system MCSI_simulation_2024_HDL_Coder_test/SPWM_3mod_hdl/tabla_spwm_g2/Decoder ==
  note: LSB
  b2 : Inport
  b1 : Inport  Port=2
  b0 (LSB) : Inport  Port=3
  Logical Operator{,1..7} (8 alike) : Logic  Inputs=3  IconShape=distinctive  AllPortsSameDT=off  OutDataTypeStr=boolean
  Logical Operator10 : Logic  Operator=NOT  IconShape=distinctive  AllPortsSameDT=off  OutDataTypeStr=boolean
  Logical Operator8 : Logic  Operator=NOT  IconShape=distinctive  AllPortsSameDT=off  OutDataTypeStr=boolean
  Logical Operator9 : Logic  Operator=NOT  IconShape=distinctive  AllPortsSameDT=off  OutDataTypeStr=boolean
  Out1 : Outport
  Out2 : Outport  Port=2
  Out3 : Outport  Port=3
  Out4 : Outport  Port=4
  Out5 : Outport  Port=5
  Out6 : Outport  Port=6
  Out7 : Outport  Port=7
  Out8 : Outport  Port=8
  wires:
  Logical Operator9/1 -> Logical Operator5/2, Logical Operator4/2, Logical Operator1/2, Logical Operator/2
  Logical Operator5/1 -> Out6/1
  Logical Operator1/1 -> Out2/1
  Logical Operator10/1 -> Logical Operator3/3, Logical Operator2/3, Logical Operator/3, Logical Operator1/3
  Logical Operator/1 -> Out1/1
  Logical Operator8/1 -> Logical Operator6/1, Logical Operator4/1, Logical Operator2/1, Logical Operator/1
  b2/1 -> Logical Operator4/3, Logical Operator5/3, Logical Operator7/3, Logical Operator6/3, Logical Operator10/1
  b0 (LSB)/1 -> Logical Operator7/1, Logical Operator5/1, Logical Operator3/1, Logical Operator1/1, Logical Operator8/1
  Logical Operator7/1 -> Out8/1
  b1/1 -> Logical Operator3/2, Logical Operator2/2, Logical Operator7/2, Logical Operator6/2, Logical Operator9/1
  Logical Operator4/1 -> Out5/1
  Logical Operator6/1 -> Out7/1
  Logical Operator3/1 -> Out4/1
  Logical Operator2/1 -> Out3/1

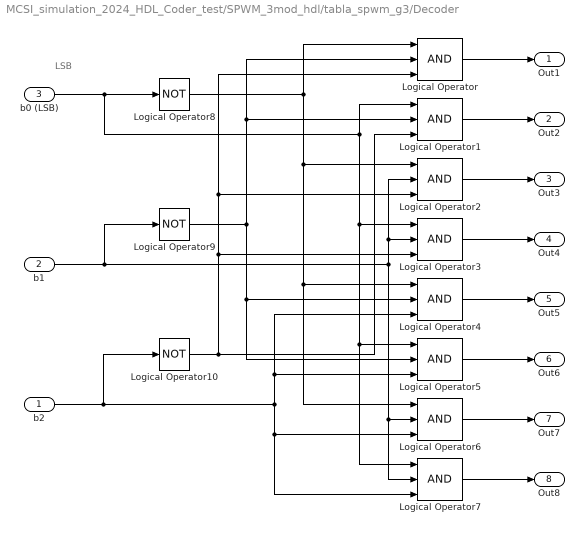
== system MCSI_simulation_2024_HDL_Coder_test/SPWM_3mod_hdl/tabla_spwm_g3/Decoder ==
  note: LSB
  b2 : Inport
  b1 : Inport  Port=2
  b0 (LSB) : Inport  Port=3
  Logical Operator{,1..7} (8 alike) : Logic  Inputs=3  IconShape=distinctive  AllPortsSameDT=off  OutDataTypeStr=boolean
  Logical Operator10 : Logic  Operator=NOT  IconShape=distinctive  AllPortsSameDT=off  OutDataTypeStr=boolean
  Logical Operator8 : Logic  Operator=NOT  IconShape=distinctive  AllPortsSameDT=off  OutDataTypeStr=boolean
  Logical Operator9 : Logic  Operator=NOT  IconShape=distinctive  AllPortsSameDT=off  OutDataTypeStr=boolean
  Out1 : Outport
  Out2 : Outport  Port=2
  Out3 : Outport  Port=3
  Out4 : Outport  Port=4
  Out5 : Outport  Port=5
  Out6 : Outport  Port=6
  Out7 : Outport  Port=7
  Out8 : Outport  Port=8
  wires:
  Logical Operator9/1 -> Logical Operator5/2, Logical Operator4/2, Logical Operator1/2, Logical Operator/2
  Logical Operator5/1 -> Out6/1
  Logical Operator1/1 -> Out2/1
  Logical Operator10/1 -> Logical Operator3/3, Logical Operator2/3, Logical Operator/3, Logical Operator1/3
  Logical Operator/1 -> Out1/1
  Logical Operator8/1 -> Logical Operator6/1, Logical Operator4/1, Logical Operator2/1, Logical Operator/1
  b2/1 -> Logical Operator4/3, Logical Operator5/3, Logical Operator7/3, Logical Operator6/3, Logical Operator10/1
  b0 (LSB)/1 -> Logical Operator7/1, Logical Operator5/1, Logical Operator3/1, Logical Operator1/1, Logical Operator8/1
  Logical Operator7/1 -> Out8/1
  b1/1 -> Logical Operator3/2, Logical Operator2/2, Logical Operator7/2, Logical Operator6/2, Logical Operator9/1
  Logical Operator4/1 -> Out5/1
  Logical Operator6/1 -> Out7/1
  Logical Operator3/1 -> Out4/1
  Logical Operator2/1 -> Out3/1
